simulink model "fromscratch"  (R2022b)
settings: Solver=VariableStepAuto  StartTime=0.0  StopTime=10.0  RelTol=1e-3
values from neighbouring files (symbols this model uses):
  gimbal_offset_pitch = (randn*0.0174533*0.1)    [MonteCarlo.m]
  gimbal_offset_yaw = (randn*0.0174533*0.1)    [MonteCarlo.m]
  Imatrix = [0.06 0 0; 0 0.06 0; 0 0 0.04]    [MonteCarlo.m]
  torquemultiplier = (randn*0.0174533*15)    [MonteCarlo.m]
undefined symbols (not defined in the file or in its folder): DiscIntNeverNeededParam, sigbuilder_block
libraries: simulink x2, shared6dof x1
settings Model: Creator=Freddie  LastModifiedBy=Freddie

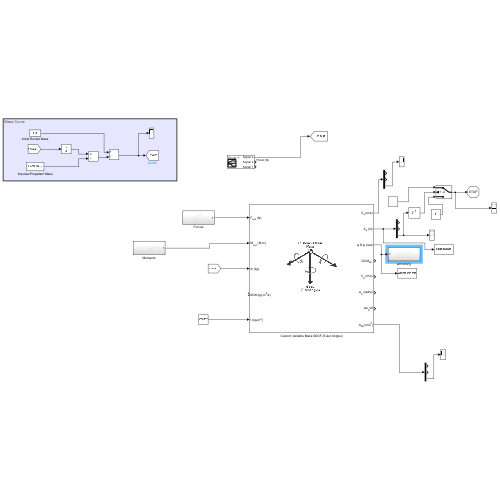
[thumbnail: Simulink's stored preview of the top-level diagram]
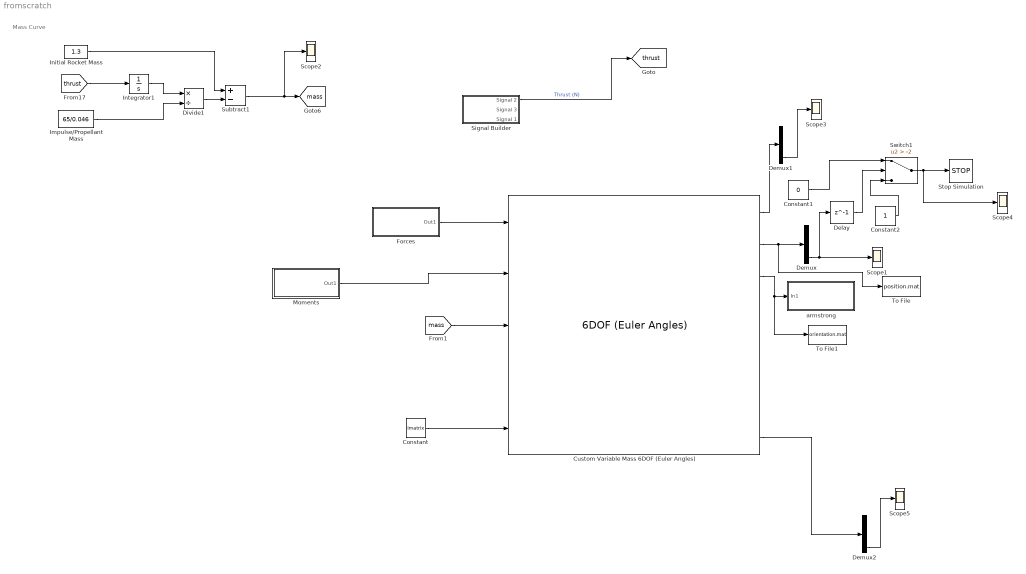
== system fromscratch ==
  note: Mass Curve
  Constant : Constant  Value=Imatrix
  Constant1 : Constant  Value=0
  Constant2 : Constant
  Custom Variable Mass 6DOF (Euler Angles) : shared6dof/6DOF (Euler Angles)  units=Metric (MKS)  mtype=Custom Variable  rep=Euler Angles  xme_0=[0 0 0]  Vm_0=[0 0 0]  eul_0=[0 0 0]  pm_0=[0 0 0]  mass_0=1.0  mass_e=0.5  mass_f=2.0  inertia=eye(3)  inertia_e=eye(3)  inertia_f=2*eye(3)  k_quat=1.0  vre_flag=off  abi_flag=off  aMode=0  xme_statename=''  Vm_statename=''  eul_statename=''  quat_statename=''  pm_statename=''  mass_statename=''
      settings: LibrarySourceBlock=aerolib6dof2/Custom Variable Mass 6DOF (Euler Angles)
  Delay : Delay  DelayLength=1  InitialCondition=0
  Demux : Demux  Outputs=3
  Demux1 : Demux  Outputs=3
  Demux2 : Demux  Outputs=3
  Divide1 : Product  Inputs=*/
  Forces : Subsystem
  Impulse/Propellant Mass : Constant  Value=65/0.046
  Initial Rocket Mass : Constant  Value=1.3
  Integrator1 : Integrator
  Moments : Subsystem
  Scope{1..5} (5 alike) : Scope
  Signal Builder : Subsystem  Tag=STV Subsys  LoadFcn=sigbuilder_block('load');  StartFcn=sigbuilder_block('start');  StopFcn=sigbuilder_block('stop');  ClipboardFcn=sigbuilder_block('clipboard');  mask(Sigbuilder block){tuvar=[0:10]}
      mask help: Simulink:masks:SigbuilderBlock_MD
      mask init:
      | if ~strcmp(get_param(bdroot(gcbh),'SimulationStatus'),'stopped') tuvar = sigbuilder_block('maskInit'); end
      settings: CopyFcn=sigbuilder_block('copy');  DeleteFcn=sigbuilder_block('delete');  ModelCloseFcn=sigbuilder_block('modelClose');  PreSaveFcn=sigbuilder_block('preSave');  PauseFcn=sigbuilder_block('pause');  ContinueFcn=sigbuilder_block('continue');  NameChangeFcn=sigbuilder_block('namechange');  OpenFcn=sigbuilder_block('open',[437.6 199.2 550.4 400 ]);  CloseFcn=sigbuilder_block('close');
      mask Display: plot(0, 0, 100, 100,[2, 2, 32, 32, 2], [68, 8, 8, 68, 68],[32, 2], [38, 38], [32, 19, 2],[53, 60, 44], [32, 17, 17, 2],[16, 16, 31, 31]);txt = getActiveGroup(gcbh);text(2, 100, txt,'verticalAlignment', 'top');
  Stop Simulation : Stop
  Subtract1 : Sum  Inputs=+-
  Switch1 : Switch  Criteria=u2 > Threshold  Threshold=-2  SaturateOnIntegerOverflow=off  InputSameDT=off
  To File : ToFile  Filename=position.mat  MatrixName=Position  SampleTime=0.001
  To File1 : ToFile  Filename=orientation.mat  MatrixName=Orientation  SampleTime=0.001
  armstrong : Subsystem
  tag scope: mass=global, thrust=global
  wires:
  Moments/1(Out1) -> Custom Variable Mass 6DOF (Euler Angles)/2
  Custom Variable Mass 6DOF (Euler Angles)/3 -> To File1/1, armstrong/1(In1)
  Custom Variable Mass 6DOF (Euler Angles)/2 -> To File/1, Demux/1
  Forces/1(Out1) -> Custom Variable Mass 6DOF (Euler Angles)/1
  Signal Builder/1(Signal 2) -> [thrust]  "Thrust (N)"
  Divide1/1 -> Subtract1/2
  Integrator1/1 -> Divide1/1
  [thrust] -> Integrator1/1
  Initial Rocket Mass/1 -> Subtract1/1
  Subtract1/1 -> Scope2/1, [mass]
  Impulse/Propellant Mass/1 -> Divide1/2
  [mass] -> Custom Variable Mass 6DOF (Euler Angles)/3
  Demux/3 -> Scope1/1, Delay/1
  Constant/1 -> Custom Variable Mass 6DOF (Euler Angles)/5
  Constant1/1 -> Switch1/1
  Switch1/1 -> Scope4/1, Stop Simulation/1
  Constant2/1 -> Switch1/3
  Delay/1 -> Switch1/2
  Custom Variable Mass 6DOF (Euler Angles)/1 -> Demux1/1
  Demux1/3 -> Scope3/1
  Demux2/3 -> Scope5/1
  Custom Variable Mass 6DOF (Euler Angles)/8 -> Demux2/1

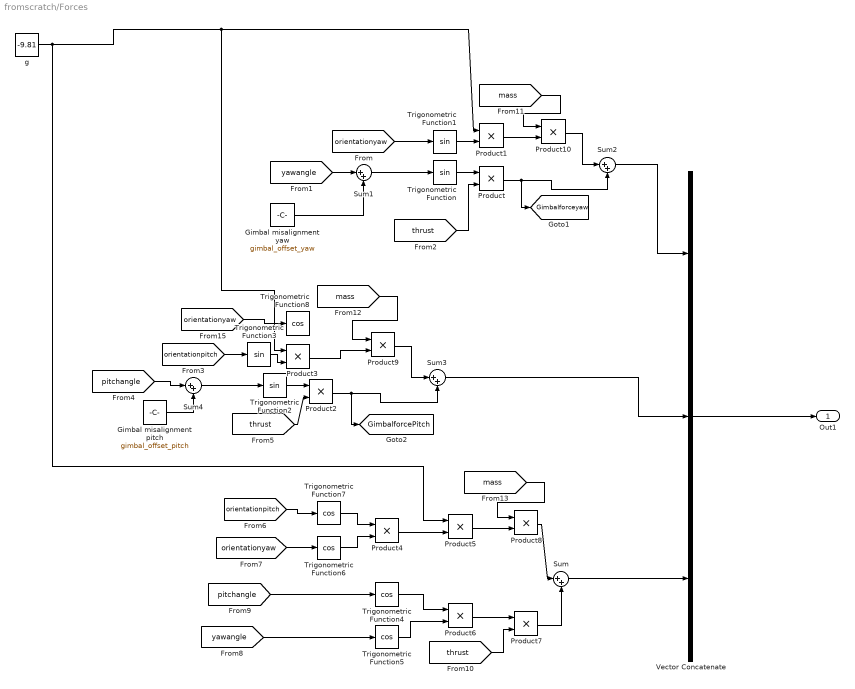
== system fromscratch/Forces ==
  Gimbal misalignment pitch : Constant  Value=gimbal_offset_pitch
  Gimbal misalignment yaw : Constant  Value=gimbal_offset_yaw
  Product{,1..10} (11 alike) : Product
  Sum{,1..4} (5 alike) : Sum  Inputs=|++
  Trigonometric Function{,1..3} (4 alike) : Trigonometry
  Trigonometric Function{4..8} (5 alike) : Trigonometry  Operator=cos
  Vector Concatenate : Concatenate  NumInputs=3
  g : Constant  Value=-9.81
  Out1 : Outport
  tag scope: GimbalforcePitch=global, Gimbalforceyaw=global
  wires:
  Trigonometric Function/1 -> Product/1
  g/1 -> Product5/1, Product3/1, Product1/1
  Trigonometric Function1/1 -> Product1/2
  Sum2/1 -> Vector Concatenate/1
  Product/1 -> [Gimbalforceyaw], Sum2/2
  [thrust] -> Product/2
  [orientationyaw] -> Trigonometric Function1/1
  Vector Concatenate/1 -> Out1/1
  [orientationpitch] -> Trigonometric Function3/1
  [thrust] -> Product2/2
  Trigonometric Function3/1 -> Product3/2
  Product2/1 -> [GimbalforcePitch], Sum3/2
  Trigonometric Function2/1 -> Product2/1
  Sum3/1 -> Vector Concatenate/2
  [orientationpitch] -> Trigonometric Function7/1
  [orientationyaw] -> Trigonometric Function6/1
  Trigonometric Function7/1 -> Product4/1
  Trigonometric Function6/1 -> Product4/2
  Product4/1 -> Product5/2
  [pitchangle] -> Trigonometric Function4/1
  [yawangle] -> Trigonometric Function5/1
  Trigonometric Function4/1 -> Product6/1
  Trigonometric Function5/1 -> Product6/2
  Sum/1 -> Vector Concatenate/3
  [yawangle] -> Sum1/1
  Sum1/1 -> Trigonometric Function/1
  Gimbal misalignment yaw/1 -> Sum1/2
  Sum4/1 -> Trigonometric Function2/1
  [pitchangle] -> Sum4/1
  Gimbal misalignment pitch/1 -> Sum4/2
  Product6/1 -> Product7/1
  Product7/1 -> Sum/2
  [thrust] -> Product7/2
  Product5/1 -> Product8/2
  Product8/1 -> Sum/1
  Product9/1 -> Sum3/1
  Product1/1 -> Product10/2
  Product10/1 -> Sum2/1
  [mass] -> Product9/1
  [mass] -> Product10/1
  [mass] -> Product8/1
  Product3/1 -> Product9/2
  [orientationyaw] -> Trigonometric Function8/1

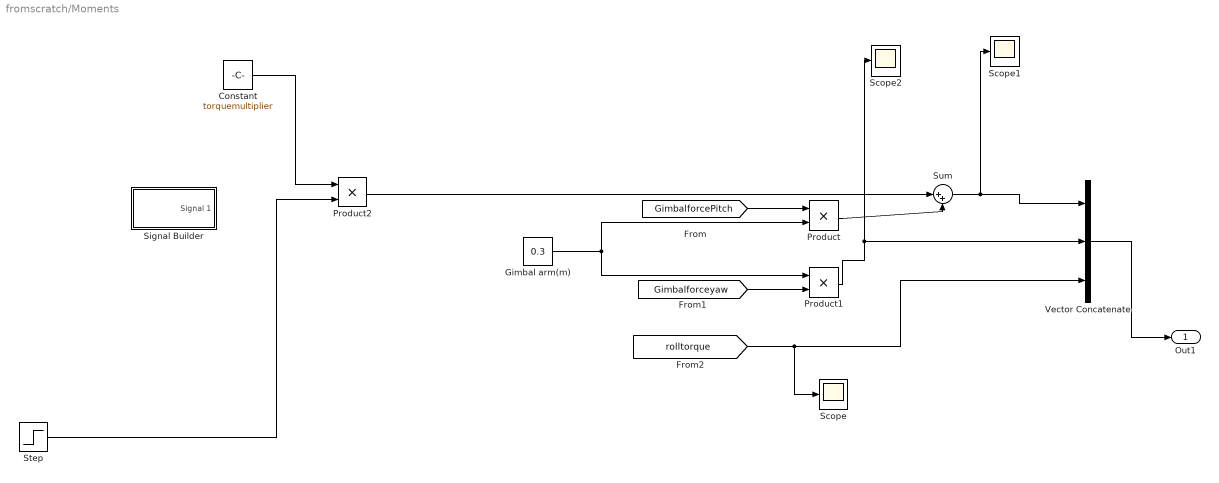
== system fromscratch/Moments ==
  Constant : Constant  Value=torquemultiplier
  Gimbal arm(m) : Constant  Value=0.3
  Product : Product
  Product1 : Product
  Product2 : Product
  Scope : Scope
  Scope1 : Scope
  Scope2 : Scope
  Signal Builder : Subsystem  Tag=STV Subsys  LoadFcn=sigbuilder_block('load');  StartFcn=sigbuilder_block('start');  StopFcn=sigbuilder_block('stop');  ClipboardFcn=sigbuilder_block('clipboard');  mask(Sigbuilder block){tuvar=[0:10]}
      mask help: Simulink:masks:SigbuilderBlock_MD
      mask init:
      | if ~strcmp(get_param(bdroot(gcbh),'SimulationStatus'),'stopped') tuvar = sigbuilder_block('maskInit'); end
      settings: CopyFcn=sigbuilder_block('copy');  DeleteFcn=sigbuilder_block('delete');  ModelCloseFcn=sigbuilder_block('modelClose');  PreSaveFcn=sigbuilder_block('preSave');  PauseFcn=sigbuilder_block('pause');  ContinueFcn=sigbuilder_block('continue');  NameChangeFcn=sigbuilder_block('namechange');  OpenFcn=sigbuilder_block('open',[437.6 199.2 550.4 400 ]);  CloseFcn=sigbuilder_block('close');
      mask Display: plot(0, 0, 100, 100,[2, 2, 32, 32, 2], [68, 8, 8, 68, 68],[32, 2], [38, 38], [32, 19, 2],[53, 60, 44], [32, 17, 17, 2],[16, 16, 31, 31]);txt = getActiveGroup(gcbh);text(2, 100, txt,'verticalAlignment', 'top');
  Step : Step  Time=0.33  Before=1  After=0  SampleTime=0
  Sum : Sum  Inputs=|++
  Vector Concatenate : Concatenate  NumInputs=3
  Out1 : Outport
  wires:
  [GimbalforcePitch] -> Product/1
  [Gimbalforceyaw] -> Product1/2
  Gimbal arm(m)/1 -> Product/2, Product1/1
  [rolltorque] -> Scope/1, Vector Concatenate/3
  Product1/1 -> Vector Concatenate/2, Scope2/1
  Vector Concatenate/1 -> Out1/1
  Step/1 -> Product2/2
  Constant/1 -> Product2/1
  Product/1 -> Sum/2
  Sum/1 -> Scope1/1, Vector Concatenate/1
  Product2/1 -> Sum/1

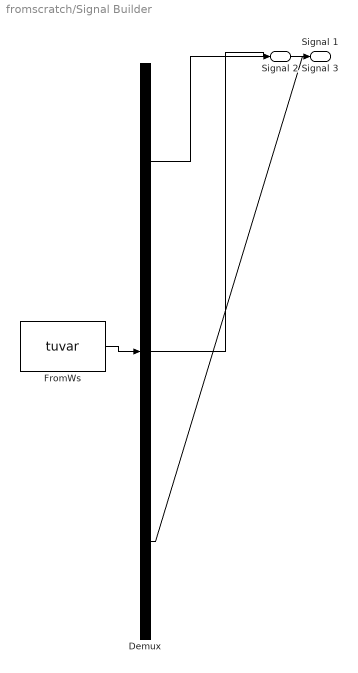
== system fromscratch/Signal Builder ==
  Demux : Demux  Tag=STV Demux  Outputs=3
      settings: DisplayOption=none
  FromWs : FromWorkspace  Tag=STV FromWs  VariableName=tuvar
      SigBuilderData=|
      | common.afterFinalStr = 'Extrapolate'
      | common.sampleTime = 0
      | dataSet.timeRange = [0 100]
      | dataSet.name = 'Group 1'
      | sbobj.Groups.Name = 'Group 1'
      | sbobj.Groups.Signals(1).Name = 'Signal 2'
      | sbobj.Groups.Signals(1).XData = [0 0.014 0.075 0.157 0.293 0.382 0.45 0.539 0.614 0.662 0.771 0.948 0.996 1.078 1.187 1.289 1.337 1.412 1.474 1.515 1.542 1.706 1.938 2.101 2.129 2.251 2.402 2.64 2.961 3.31 100]
      | sbobj.Groups.Signals(1).YData = [11.527 11.527 20.126 26.572 29.113 30.278 29.69 30.667 30.089 31.15 30.478 29.89 28.714 28.136 27.738 26.761 26.96 25.984 25.008 26.173 24.808 22.856 20.903 18.173 19.338 16.21 13.48 8.791 3.32 0 0]
      | sbobj.Groups.Signals(2).Name = 'Signal 3'
      | sbobj.Groups.Signals(2).XData = [0 3.31 100]
      | sbobj.Groups.Signals(2).YData = [1.3 1.254 1.254]
      | sbobj.Groups.Signals(3).Name = 'Signal 1'
      | sbobj.Groups.Signals(3).XData = [0 0.024 0.066 0.138 0.246 0.426 1.218 2.082 3.306 5.322 6.978 8.632 25 100]
      | sbobj.Groups.Signals(3).YData = [0.3704 0.3704 0.8746 4.5044 12.4 17.5 16.5 17.5 16.5 18.5 16 15.5 17.5 7]
      | sbobj.Groups.TimeRange = [0 100]
  Signal 2 : Outport  Tag=STV Outport
  Signal 3 : Outport  Tag=STV Outport  Port=2
  Signal 1 : Outport  Tag=STV Outport  Port=3
  wires:
  FromWs/1 -> Demux/1
  Demux/1 -> Signal 2/1
  Demux/2 -> Signal 3/1
  Demux/3 -> Signal 1/1

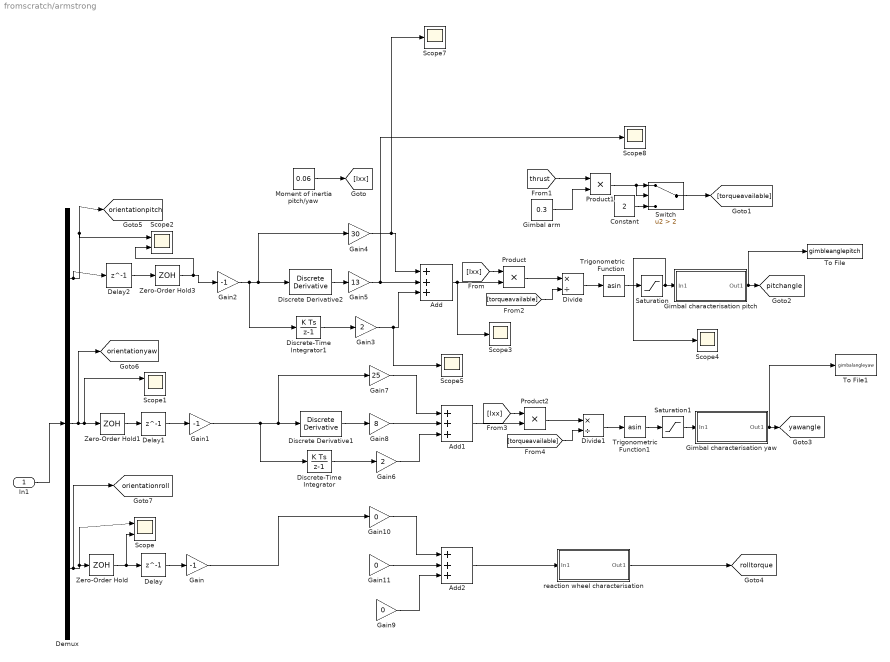
== system fromscratch/armstrong ==
  In1 : Inport
  Add : Sum  Inputs=+++
  Add1 : Sum  Inputs=+++
  Add2 : Sum  Inputs=+++
  Constant : Constant  Value=2
  Delay : Delay  DelayLength=1  InitialCondition=0
  Delay1 : Delay  DelayLength=1  InitialCondition=0
  Delay2 : Delay  DelayLength=1  InitialCondition=0
  Demux : Demux  Outputs=3
  Discrete Derivative1 : simulink/Discrete/Discrete Derivative  gainval=1.0  ICPrevScaledInput=0.0  OutMin=[]  OutMax=[]  OutDataType=fixdt(1, 16)  OutScaling=2^-10  DoSatur=off
  Discrete Derivative2 : simulink/Discrete/Discrete Derivative  gainval=1.0  ICPrevScaledInput=0.0  OutMin=[]  OutMax=[]  OutDataType=fixdt(1, 16)  OutScaling=2^-10  DoSatur=off
  Discrete-Time Integrator : DiscreteIntegrator  SampleTime=-1  ICPrevOutput=DiscIntNeverNeededParam  ICPrevScaledInput=DiscIntNeverNeededParam
  Discrete-Time Integrator1 : DiscreteIntegrator  SampleTime=-1  ICPrevOutput=DiscIntNeverNeededParam  ICPrevScaledInput=DiscIntNeverNeededParam
  Divide : Product  Inputs=*/
  Divide1 : Product  Inputs=*/
  Gain : Gain  Gain=-1
  Gain1 : Gain  Gain=-1
  Gain10 : Gain  Gain=0
  Gain11 : Gain  Gain=0
  Gain2 : Gain  Gain=-1
  Gain3 : Gain  Gain=2
  Gain4 : Gain  Gain=30
  Gain5 : Gain  Gain=13
  Gain6 : Gain  Gain=2
  Gain7 : Gain  Gain=25
  Gain8 : Gain  Gain=8
  Gain9 : Gain  Gain=0
  Gimbal arm : Constant  Value=0.3
  Gimbal characterisation pitch : Subsystem
  Gimbal characterisation yaw : Subsystem
  Moment of inertia pitch/yaw : Constant  Value=0.06
  Product : Product
  Product1 : Product
  Product2 : Product
  Saturation : Saturate  UpperLimit=0.139626  LowerLimit=-0.139626
  Saturation1 : Saturate  UpperLimit=0.139626  LowerLimit=-0.139626
  Scope : Scope  NumInputPorts=2
  Scope1 : Scope  NumInputPorts=2
  Scope2 : Scope  NumInputPorts=2
  Scope{3..5,7..8} (5 alike) : Scope
  Switch : Switch  Criteria=u2 > Threshold  Threshold=2  SaturateOnIntegerOverflow=off  InputSameDT=off
  To File : ToFile  Filename=gimbleanglepitch  MatrixName=anglep  SampleTime=0.001
  To File1 : ToFile  Filename=gimbalangleyaw  MatrixName=angley  SampleTime=0.001
  Trigonometric Function : Trigonometry  Operator=asin  OutputSignalType=real
  Trigonometric Function1 : Trigonometry  Operator=asin  OutputSignalType=real
  Zero-Order Hold : ZeroOrderHold  SampleTime=-1
  Zero-Order Hold1 : ZeroOrderHold  SampleTime=-1
  Zero-Order Hold3 : ZeroOrderHold  SampleTime=0.01
  reaction wheel characterisation : Subsystem
  tag scope: orientationpitch=global, orientationroll=global, orientationyaw=global, pitchangle=global, rolltorque=global, yawangle=global
  wires:
  In1/1 -> Demux/1
  Demux/3 -> [orientationroll], Scope/1, Zero-Order Hold/1
  Zero-Order Hold/1 -> Scope/2, Delay/1
  Delay/1 -> Gain/1
  Demux/2 -> [orientationyaw], Zero-Order Hold1/1, Scope1/1
  Demux/1 -> Delay2/1, Scope2/1, [orientationpitch]
  Moment of inertia pitch/yaw/1 -> [Ixx]
  Gain5/1 -> Scope8/1, Add/2
  Gain4/1 -> Scope7/1, Add/1
  Gain3/1 -> Scope5/1, Add/3
  Add/1 -> Scope3/1, Product/2
  [Ixx] -> Product/1
  Product/1 -> Divide/1
  [thrust] -> Product1/1
  Gimbal arm/1 -> Product1/2
  Product1/1 -> Switch/2, Switch/1
  Constant/1 -> Switch/3
  Switch/1 -> [torqueavailable]
  [torqueavailable] -> Divide/2
  Divide/1 -> Trigonometric Function/1
  Trigonometric Function/1 -> Saturation/1
  Saturation/1 -> Scope4/1, Gimbal characterisation pitch/1(In1)
  Gimbal characterisation pitch/1(Out1) -> To File/1, [pitchangle]
  Gimbal characterisation yaw/1(Out1) -> To File1/1, [yawangle]
  [torqueavailable] -> Divide1/2
  Gain8/1 -> Add1/2
  Gain6/1 -> Add1/3
  Saturation1/1 -> Gimbal characterisation yaw/1(In1)
  Gain7/1 -> Add1/1
  [Ixx] -> Product2/1
  Add1/1 -> Product2/2
  Divide1/1 -> Trigonometric Function1/1
  Product2/1 -> Divide1/1
  Trigonometric Function1/1 -> Saturation1/1
  Gain11/1 -> Add2/2
  Gain9/1 -> Add2/3
  Gain/1 -> Gain10/1
  Gain10/1 -> Add2/1
  Add2/1 -> reaction wheel characterisation/1(In1)
  reaction wheel characterisation/1(Out1) -> [rolltorque]
  Zero-Order Hold3/1 -> Scope2/2, Gain2/1
  Delay2/1 -> Zero-Order Hold3/1
  Delay1/1 -> Gain1/1
  Zero-Order Hold1/1 -> Delay1/1
  Discrete-Time Integrator/1 -> Gain6/1
  Discrete-Time Integrator1/1 -> Gain3/1
  Gain2/1 -> Discrete-Time Integrator1/1, Discrete Derivative2/1, Gain4/1
  Discrete Derivative1/1 -> Gain8/1
  Gain1/1 -> Discrete-Time Integrator/1, Discrete Derivative1/1, Gain7/1
  Discrete Derivative2/1 -> Gain5/1

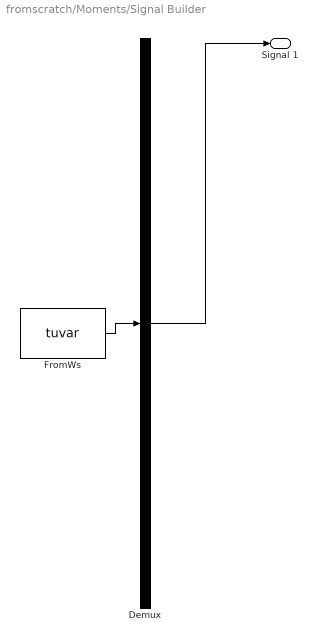
== system fromscratch/Moments/Signal Builder ==
  Demux : Demux  Tag=STV Demux  Outputs=1
      settings: DisplayOption=none
  FromWs : FromWorkspace  Tag=STV FromWs  VariableName=tuvar
      SigBuilderData=|
      | common.afterFinalStr = 'Extrapolate'
      | common.sampleTime = 0
      | dataSet.timeRange = [0 10]
      | dataSet.name = 'Group 1'
      | sbobj.Groups.Name = 'Group 1'
      | sbobj.Groups.Signals.Name = 'Signal 1'
      | sbobj.Groups.Signals.XData = [0 6 6 10]
      | sbobj.Groups.Signals.YData = [1.015 1 0 0]
  Signal 1 : Outport  Tag=STV Outport
  wires:
  Demux/1 -> Signal 1/1
  FromWs/1 -> Demux/1

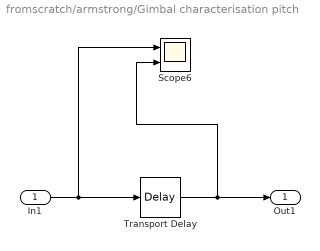
== system fromscratch/armstrong/Gimbal characterisation pitch ==
  In1 : Inport
  Scope6 : Scope  NumInputPorts=2
  Transport Delay : TransportDelay  DelayTime=0.03
  Out1 : Outport
  wires:
  In1/1 -> Scope6/1, Transport Delay/1
  Transport Delay/1 -> Scope6/2, Out1/1

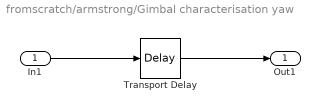
== system fromscratch/armstrong/Gimbal characterisation yaw ==
  In1 : Inport
  Transport Delay : TransportDelay  DelayTime=0.03
  Out1 : Outport
  wires:
  In1/1 -> Transport Delay/1
  Transport Delay/1 -> Out1/1

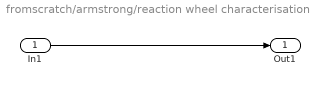
== system fromscratch/armstrong/reaction wheel characterisation ==
  In1 : Inport
  Out1 : Outport
  wires:
  In1/1 -> Out1/1
